simulink model "model_satelita"  (R2022b)
settings: Solver=ode4  StartTime=0.0  StopTime=10.0  FixedStep=2^(-7)  RelTol=1e-3
libraries: simulink x1
settings Model: Creator=bm50345  LastModifiedBy=bm50345

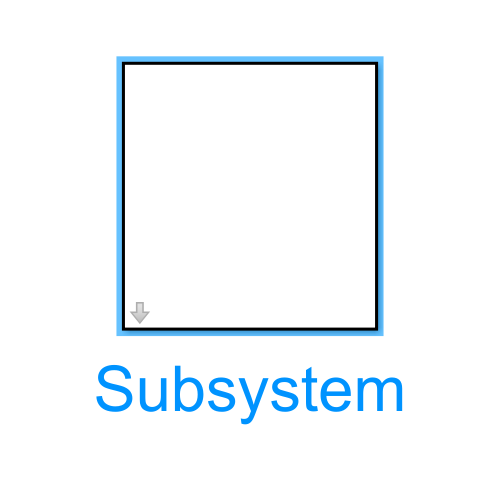
[thumbnail: Simulink's stored preview of the top-level diagram]
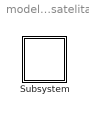
== system model_satelita ==
  Subsystem : Subsystem  mask{x0=0, y0=5, vx0=10, vy0=0, m=200, r=2, g=9.81, rs=0.2}

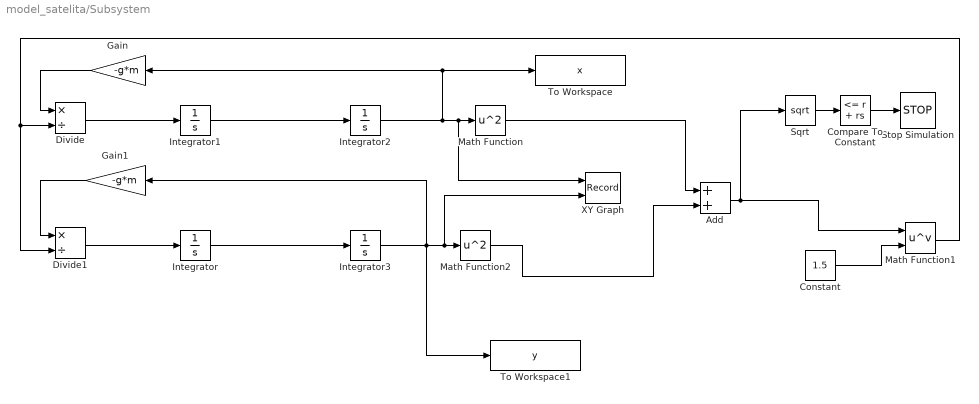
== system model_satelita/Subsystem ==
  Add : Sum
  Compare To Constant : simulink/Logic and Bit Operations/Compare To Constant  relop=<=  const=r + rs  OutDataTypeStr=boolean
  Constant : Constant  Value=1.5
  Divide : Product  Inputs=*/
  Divide1 : Product  Inputs=*/
  Gain : Gain  Gain=-g*m
  Gain1 : Gain  Gain=-g*m
  Integrator : Integrator  InitialCondition=vy0
  Integrator1 : Integrator  InitialCondition=vx0
  Integrator2 : Integrator  InitialCondition=x0
  Integrator3 : Integrator  InitialCondition=y0
  Math Function : Math  Operator=square
  Math Function1 : Math  Operator=pow
  Math Function2 : Math  Operator=square
  Sqrt : Sqrt
  Stop Simulation : Stop
  To Workspace : ToWorkspace  VariableName=x  SampleTime=-1
  To Workspace1 : ToWorkspace  VariableName=y  SampleTime=-1
  XY Graph : Record  FileSettingsInternal="{\"entries\":[{\"content\":{\"excelSettings\":{\"content\":{},\"type\":\"Streamout.ExcelSettings\"}},\"type\":\"Streamout.FileSettingStorage\",\"uuid\":\"ede3ea44-2cc3-48fe-8127-2c78db362564\"}],\"packageUris\":[\"http://schema.mathworks.com/mf0/streamout_blocks/R2020a\"],\"version\":\"1.0\"}"  Layout=[1 1]  SignalsInternal="{\"entries\":[{\"content\":{\"signals\":[{\"content\":{\"blockPath\":[\"model_satelita/Subsystem/XY Graph\"],\"channel\":[],\"dimensions\":[1],\"domain\":\"model_satelita/Subsystem/XY Graph\",\"lineColor\":\"#a2142f\",\"plots\":[1],\"port\":1,\"sid\":[\"\"],\"signalID\":622,\"signalName\":\"Integrator2\"},\"type\":\"RecordBlkView.Signal\",\"uuid\":\"bba46acf-165e-4a22-aa6f-08fa4328cde0\"},{\"content\":{\"blockPath\":[\"model_satelita/Subsystem/XY Graph\"],\"channel\":[],\"dimensions\":[1],\"domain\":\"model_satelita/Subsystem/XY Graph\",\"lineColor\":\"#139fff\",\"plots\":[1],\"port\":2,\"sid\":[\"\"],\"signalID\":626,\"signalName\":\"Integrator3\"},\"type\":\"RecordBlkView.Signal\",\"uuid\":\"8cd6c7d5-cccc-4d94-9c40-a73258f0501e\"}]},\"type\":\"RecordBlkView.InputSignals\",\"uuid\":\"19a67a69-3c85-4e24-8b6b-3369a4e85cb8\"}],\"packageUris\":[\"http://schema.mathworks.com/mf0/streamout_blocks/R2020a\"],\"version\":\"1.0\"}"  VisualizationBindings="{\"xyplotplugin\":{\"info\":[{\"series\":[{\"bindingParametersList\":[{\"parameter\":\"X-Axis\",\"signalID\":622,\"signalName\":\"Integrator2\"},{\"parameter\":\"Y-Axis\",\"signalID\":626,\"signalName\":\"Integrator3\"}],\"seriesID\":34212}],\"subplotID\":1}]}}"  CompatibilityTag=XY
  wires:
  Math Function1/1 -> Divide1/2, Divide/2
  Math Function/1 -> Add/1
  Constant/1 -> Math Function1/2
  Math Function2/1 -> Add/2
  Add/1 -> Sqrt/1, Math Function1/1
  Integrator3/1 -> To Workspace1/1, Gain1/1, XY Graph/2, Math Function2/1
  Gain/1 -> Divide/1
  Integrator/1 -> Integrator3/1
  Integrator1/1 -> Integrator2/1
  Gain1/1 -> Divide1/1
  Divide1/1 -> Integrator/1
  Divide/1 -> Integrator1/1
  Integrator2/1 -> To Workspace/1, Gain/1, XY Graph/1, Math Function/1
  Sqrt/1 -> Compare To Constant/1
  Compare To Constant/1 -> Stop Simulation/1
